simulink model "Motor"  (Simulink 7.9)
settings: Solver=ode45  StartTime=0.0  StopTime=0.2  MaxStep=0.0000008  RelTol=1e-8
values from neighbouring files (symbols this model uses):
  J = Jm+J_last/i_getr^2    (= 1.07037741047e-06)    [DC_Motor_RI_Comp.m]
  M_Load = M_last/(i_getr*eta_getr)    (= 0.00103003721425)    [DC_Motor_RI_Comp.m]
  Mo = Io*Psi    (= 0.000558650326277)    [DC_Motor_RI_Comp.m]    (also in Sim_Kinematik_Modelle.m = 0.00152232213911; Tol_Kinematik_Modell.m = Io.*Psi)
  P = 50    [DC_Motor_RI_Comp.m]
  Phi = w_stat*t+(wo-w_stat)*(T1*k1*(1-exp(-t/T1))+T2*k2*(1-exp(-t/T2)))    [Motor_1.m]    (also in Sim_Kinematik_Modelle.m = [Phi max(Phi)+Phi_on max(Phi)+max(Phi_on)+Phi_off])
  Ra = 6.7    [DC_Motor_RI_Comp.m]    (also in Sim_Kinematik_Modelle.m = 5.1322; Tol_Kinematik_Modell.m = Ra_20*(1+Kr*(T(T_N)-20)))
  Rc = 0.0*Ra    (= 0)    [DC_Motor_RI_Comp.m]    (also in Sim_Kinematik_Modelle.m)
  T_PWM = 1/f_PWM    (= 1.6e-05)    [DC_Motor_RI_Comp.m]    (also in Sim_Kinematik_Modelle.m = 0.005)
  Tc = 0.8*Tm    (= 0.0226483122607)    [DC_Motor_RI_Comp.m]    (also in Sim_Kinematik_Modelle.m = 0.00182524694804)
  Umax = 8*0.8    (= 6.4)    [DC_Motor_RI_Comp.m]
undefined symbols (not defined in the file or in its folder): L
settings Model: Creator=dep02378  LastModifiedBy=dep02378
settings OptimizationCC: InitFltsAndDblsToZero=on
settings DebuggingCC: FcnCallInpInsideContextMsg=Use local settings  StrictBusMsg=Warning
settings GRTTargetCC: CombineOutputUpdateFcns=off  GRTInterface=on

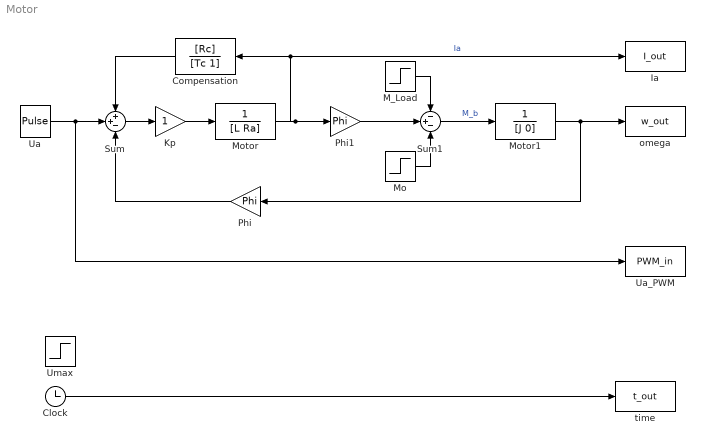
== system Motor ==
  Clock : Clock
  Compensation : TransferFcn  Numerator=[Rc]  Denominator=[Tc 1]
  Ia : ToWorkspace  VariableName=I_out  SampleTime=-1
  Kp : Gain
  M_Load : Step  Time=0.1  After=M_Load  SampleTime=0
  Mo : Step  Time=0.01  After=Mo  SampleTime=0
  Motor : TransferFcn  Denominator=[L Ra]
  Motor1 : TransferFcn  Denominator=[J 0]
  Phi : Gain  Gain=Phi
  Phi1 : Gain  Gain=Phi
  Sum : Sum  Inputs=++-
  Sum1 : Sum  Inputs=-+-
  Ua : DiscretePulseGenerator  PulseType=Time based  Amplitude=Umax  Period=T_PWM  PulseWidth=P
  Ua_PWM : ToWorkspace  VariableName=PWM_in  SampleTime=-1
  Umax : Step  Time=0.01  After=Umax  SampleTime=0
  omega : ToWorkspace  VariableName=w_out  SampleTime=-1
  time : ToWorkspace  VariableName=t_out  SampleTime=-1
  wires:
  Sum/1 -> Kp/1
  Kp/1 -> Motor/1
  Motor/1 -> Phi1/1, Compensation/1, Ia/1  "Ia"
  Clock/1 -> time/1
  Motor1/1 -> Phi/1, omega/1
  Sum1/1 -> Motor1/1  "M_b"
  Phi1/1 -> Sum1/2
  M_Load/1 -> Sum1/1
  Mo/1 -> Sum1/3
  Phi/1 -> Sum/3
  Compensation/1 -> Sum/1
  Ua/1 -> Sum/2, Ua_PWM/1
